simulink model "BD_PAR_AUTO_base_model"  (Simulink 10.3)
settings: Solver=ode1  StartTime=0.0  StopTime=max(cyc_mph(:,1))  FixedStep=1  MaxStep=1  RelTol=1e-3  AbsTol=1e-3
undefined symbols (not defined in the file): acc_dcdc_eff, acc_elec_eff, acc_elec_pwr, acc_mech_eff, acc_mech_pwr, acc_mech_trq, air_cp, amb_tmp, cs_charge_deplete_bool, cs_charge_trq, cs_electric_decel_spd, cs_electric_launch_spd_hi, cs_electric_launch_spd_lo, cs_hi_soc, cs_lo_soc, cs_min_trq_frac, cs_off_trq_frac, cyc_avg_time, cyc_cargo_mass, cyc_elevation_init, cyc_filter_bool, cyc_grade, cyc_mph, enable_sim_stop_distance, enable_sim_stop_max_spd, enable_sim_stop_speed, enable_sim_stop_time, enable_stop, enable_stop_fc, ess_cap_scale, ess_coulombic_eff, ess_init_soc, ess_max_ah_cap, ess_max_volts, ess_min_volts, ess_mod_airflow, ess_mod_cp, ess_mod_init_tmp, ess_module_mass, ess_module_num, ess_on, ess_r_chg, ess_r_dis, ess_res_scale_coef, ess_res_scale_fun, ess_set_tmp, ess_soc, ess_th_calc, ess_th_res_off, ess_th_res_on, ess_tmp, ess_voc, ex_calc, ex_cat_co_frac, ex_cat_ext_cp, ex_cat_ext_emisv, ex_cat_ext_init_tmp, ex_cat_ext_mass, ex_cat_ext_sarea, ex_cat_hc_frac ... (+168)
(part 5 of 15)

== system BD_PAR_AUTO_base_model/<vc> par auto/gearbox control for use w/ AT/est. engine trq and spd ==
  prev gear number : Inport
  " prev eta_gb" : Inport  Port=2
  gb_trq_out_r : Inport  Port=3
  gb_spd_out_r : Inport  Port=4
  Block NOTES : Subsystem
      mask Display: disp('Block\nNOTES')
  Constant2 : Constant  Value=[1 1]
  Constant5 : Constant  Value=0
  Demux : Demux  Outputs=2
      settings: DisplayOption=none
  K_adv : Subsystem
  Logical Operator : Logic
  Logical Operator1 : Logic  Operator=NOT  Inputs=1
  Memory : Memory
  Mux1 : Mux  Inputs=2
  Mux2 : Mux  Inputs=2
  Relational Operator1 : RelationalOperator  Operator=>  RndMeth=Nearest  InputSameDT=on
  SR Look-Up Table SR=wout/win : Lookup  InputValues=htc_k_adv  Table=htc_sr
  Saturation1 : Saturate  UpperLimit=1  LowerLimit=0.7
  Saturation2 : Saturate  UpperLimit=inf  LowerLimit=0
  Switch : Switch  Threshold=eps
  TR Look-Up Table TR=Tout/Tin : Lookup  InputValues=htc_k_adv  Table=htc_tr
  TR,SR : Mux  Inputs=2
  gear ratio1 : Lookup  InputValues=[1:length(gb_ratio)]  Table=gb_ratio
  ~eng trq and spd : Product  Inputs=*/  InputSameDT=on  RndMeth=Zero  SaturateOnIntegerOverflow=on  OutDataTypeStr=Inherit: Same as first input
  ~gb_spd_in_r : Product  InputSameDT=on  RndMeth=Zero  SaturateOnIntegerOverflow=on  OutDataTypeStr=Inherit: Same as first input
  ~gb_trq_in_r : Product  Inputs=//*  InputSameDT=on  RndMeth=Zero  SaturateOnIntegerOverflow=on  OutDataTypeStr=Inherit: Same as first input
  est eng trq (Nm) : Outport
  est eng spd (rad/s) : Outport  Port=2
  gb_spd_in_est (rad/s)1 : Outport  Port=3
  wires:
  gb_trq_out_r/1 -> ~gb_trq_in_r/3
  gb_spd_out_r/1 -> ~gb_spd_in_r/2
  gear ratio1/1 -> ~gb_trq_in_r/1, ~gb_spd_in_r/1
  TR,SR/1 -> Switch/1
  Constant2/1 -> Switch/3
  Switch/1 -> ~eng trq and spd/2
  " prev eta_gb"/1 -> Saturation1/1
  Saturation1/1 -> ~gb_trq_in_r/2
  Demux/2 -> Saturation2/1
  Saturation2/1 -> est eng spd (rad/s)/1
  Constant5/1 -> Relational Operator1/2
  Relational Operator1/1 -> Logical Operator/1
  prev gear number/1 -> gear ratio1/1
  Demux/1 -> est eng trq (Nm)/1
  Memory/1 -> Logical Operator1/1
  Logical Operator1/1 -> Logical Operator/2
  Logical Operator/1 -> Switch/2
  [locked_up] -> Memory/1
  Mux1/1 -> ~eng trq and spd/1
  ~eng trq and spd/1 -> Demux/1
  Mux2/1 -> K_adv/1("Req'd output trq and spd (Nm), (rad/s)")
  K_adv/1(K_adv) -> TR Look-Up Table TR=Tout/Tin/1, SR Look-Up Table SR=wout/win/1
  TR Look-Up Table TR=Tout/Tin/1 -> TR,SR/1
  SR Look-Up Table SR=wout/win/1 -> TR,SR/2
  ~gb_trq_in_r/1 -> Mux2/1, Mux1/1, Relational Operator1/1
  ~gb_spd_in_r/1 -> Mux1/2, gb_spd_in_est (rad/s)1/1, Mux2/2

== system BD_PAR_AUTO_base_model/<vc> par auto/gearbox control for use w/ AT/est. engine trq and spd assuming lockup ==
  new gear number : Inport
  " prev eta_gb" : Inport  Port=2
  gb_trq_out_r : Inport  Port=3
  gb_spd_in_est : Inport  Port=4
  Block NOTES : Subsystem
      mask Display: disp('Block\nNOTES')
  Memory : Memory  InitialCondition=gb_ratio(1)
  Saturation1 : Saturate  UpperLimit=1  LowerLimit=0.7
  Saturation2 : Saturate  UpperLimit=inf  LowerLimit=0
  gear ratio1 : Lookup  InputValues=[1:length(gb_ratio)]  Table=gb_ratio
  ~gb_spd_in_r : Product  Inputs=*/*  InputSameDT=on  RndMeth=Zero  SaturateOnIntegerOverflow=on  OutDataTypeStr=Inherit: Same as first input
  ~gb_trq_in_r : Product  Inputs=//*  InputSameDT=on  RndMeth=Zero  SaturateOnIntegerOverflow=on  OutDataTypeStr=Inherit: Same as first input
  est eng trq (Nm) : Outport
  est eng spd (rad/s) : Outport  Port=2
  wires:
  Saturation1/1 -> ~gb_trq_in_r/2
  " prev eta_gb"/1 -> Saturation1/1
  gear ratio1/1 -> ~gb_trq_in_r/1, ~gb_spd_in_r/1, Memory/1
  gb_trq_out_r/1 -> ~gb_trq_in_r/3
  new gear number/1 -> gear ratio1/1
  Saturation2/1 -> est eng spd (rad/s)/1
  Memory/1 -> ~gb_spd_in_r/2
  gb_spd_in_est/1 -> ~gb_spd_in_r/3
  ~gb_trq_in_r/1 -> est eng trq (Nm)/1
  ~gb_spd_in_r/1 -> Saturation2/1

== system BD_PAR_AUTO_base_model/<vc> par auto/gearbox control for use w/ AT/shifting1 ==
  gear number : Inport
  Constant : Constant  Value=gb_shift_delay-1e-6
  Relational Operator : RelationalOperator  Operator=<  RndMeth=Nearest  InputSameDT=on
  time since last shift : Subsystem
      mask Display: disp('time since\nlast shift')
  out_1 : Outport  InitialOutput=0
  wires:
  time since last shift/1(out_1) -> Relational Operator/1
  Constant/1 -> Relational Operator/2
  gear number/1 -> time since last shift/1(in_1)
  Relational Operator/1 -> out_1/1

== system BD_PAR_AUTO_base_model/<vc> par auto/gearbox control for use w/ AT/upshift  command ==
  prev gear number : Inport
  engine load : Inport  Port=2
  engine speed : Inport  Port=3
  Mux : Mux  Inputs=2
  Relational Operator : RelationalOperator  Operator=<  RndMeth=Nearest  InputSameDT=on
  load fraction : Subsystem  mask(Gear Selector){spd=gb_upshift_spd, load=gb_upshift_load}
      mask prompts: spd "Speeds:"; load "Load Fractions:"
      mask help:
      | This block will perform a linear interplation (extrapolation outside of bounds) to determine the shift point load fraction associated with the current gear number and speed.
      |
      | The Speeds parameter should be defined as an array of vectors containing speeds for each gear number.  The Load Fractions parameter should be defined as a array of vectors containing load fractions indexed by the speeds in the Speeds parameter for each gear number.
      mask Help:
      | Reference the base workspace variables - gb_**shift_spd and gb_**shift_load  where ** is either up for upshift conditions or dn for downshift conditions.
      | 
      | Or define the arrays as follows:
      | 
      | {[spd1 spd2 spd3 spd4]; [spd1 spd2 spd3 spd4]; ...}
      | 
      | {[load1 load2 load3 load4]; [load1 load2 load3 load4]; ...}
      | 
      | where each array contains one row for each gear in the gearbox.  Speeds should be defined in rad/s and loads as a decimal fraction.
  command : Outport  InitialOutput=0
  wires:
  load fraction/1(Out1) -> Relational Operator/2
  engine load/1 -> Relational Operator/1
  prev gear number/1 -> Mux/1
  Mux/1 -> load fraction/1(In1)
  engine speed/1 -> Mux/2
  Relational Operator/1 -> command/1

== system BD_PAR_AUTO_base_model/<vc> par auto/motor controller logic/Block NOTES ==
  note: This block models a motor/controller's logic, modulating the power input requirement as follows:
      | - enforcing the maximum current limit of the motor/controller
      | - shutting the motor off if the average speed over the time step ==0
      | - shutting the motor off if the transmission is shifting.

== system BD_PAR_AUTO_base_model/<vc> par auto/motor controller logic/Sign ==
  in_1 : Inport
  Constant : Constant  Value=0
  Relational Operator : RelationalOperator  Operator=>  RndMeth=Nearest  InputSameDT=on
  Relational Operator1 : RelationalOperator  Operator=<  RndMeth=Nearest  InputSameDT=on
  Sum : Sum  Inputs=+-  InputSameDT=on  SaturateOnIntegerOverflow=on  OutDataTypeStr=Inherit: Same as first input
  out_1 : Outport  InitialOutput=0
  wires:
  Sum/1 -> out_1/1
  Relational Operator/1 -> Sum/1
  Relational Operator1/1 -> Sum/2
  Constant/1 -> Relational Operator/2, Relational Operator1/2
  in_1/1 -> Relational Operator1/1, Relational Operator/1

== system BD_PAR_AUTO_base_model/<vc> par auto/parallel clutch control/Block NOTES ==
  note: This clutch control block determines the clutch state given the req'd clutch output torque
      | and speed (labelled as gearbox input torque and speed), and the gear number history.
      |                           conditions                                                                       clutch state
      | gear is being shifted OR (trq <~ 0 AND (engine is                                     1 == disengaged
      | clutched to avoid compression braking OR spd < idle))
      |
      | (trq >~ 0) AND (spd < launch speed) AND clutch                                       2 == slipping
      | was not engaged during previous time step
      |
      | neither of above sets of conditions are met                                          3 == engaged
      |
      | But the clutch is always disengaged when the engine is off or was off within the past 0.5 s.

== system BD_PAR_AUTO_base_model/<vc> par auto/parallel clutch control/gearbox speed estimator ==
  gb_spd_in_r if no gear change : Inport
  Block NOTES : Subsystem
      mask Display: disp('Block\nNOTES')
  Constant : Constant  Value=eps
  Constant1 : Constant  Value=0
  Constant2 : Constant
  Constant3 : Constant  Value=0.11
  Gain : Gain  Gain=0.447  SaturateOnIntegerOverflow=on  OutDataTypeStr=Inherit: Same as input  ParamDataTypeStr=Inherit: Same as input
  Logical : Logic
  Memory : Memory  InitialCondition=cyc_mph(1,2)*0.447/wh_radius*fd_ratio*gb_ratio(gb_num_init)
  Memory1 : Memory  InitialCondition=1
  Product : Product  Inputs=**/  InputSameDT=on  RndMeth=Zero  SaturateOnIntegerOverflow=on  OutDataTypeStr=Inherit: Same as first input
  Relational : RelationalOperator  Operator=>  RndMeth=Nearest  InputSameDT=on
  Relational1 : RelationalOperator  Operator=<=  RndMeth=Nearest  InputSameDT=on
  Sum : Sum  InputSameDT=on  SaturateOnIntegerOverflow=on  OutDataTypeStr=Inherit: Same as first input
  Sum1 : Sum  Inputs=-+  InputSameDT=on  SaturateOnIntegerOverflow=on  OutDataTypeStr=Inherit: Same as first input
  Switch : Switch  Threshold=eps
  Switch1 : Switch  Threshold=eps
  dt : Subsystem
  Out1 : Outport
  wires:
  Product/1 -> Switch/1
  Sum/1 -> Product/3
  Gain/1 -> Product/2
  [veh_spd_a_rec] -> Sum/1, Switch/2
  Constant1/1 -> Switch/3
  Memory/1 -> Switch1/1
  Constant/1 -> Sum/2
  [cyc_mph_r] -> Sum1/2
  [mpha] -> Gain/1, Sum1/1
  Constant2/1 -> Relational/2
  Sum1/1 -> Relational/1
  Relational/1 -> Memory1/1
  Switch/1 -> Memory/1
  Switch1/1 -> Out1/1
  gb_spd_in_r if no gear change/1 -> Switch1/3
  [gb_spd_in_a] -> Product/1
  Constant3/1 -> Relational1/2
  Relational1/1 -> Logical/2
  Memory1/1 -> Logical/1
  Logical/1 -> Switch1/2
  dt/1(Out1) -> Relational1/1

== system BD_PAR_AUTO_base_model/<vc> par auto/sim stop subsystem/Block NOTES ==
  note: This block controls the simulation stop time.  The simulation maybe
      | stop based on the achievement of a specified speed, a max speed, a time, a distance, or an engine condition.

== system BD_PAR_AUTO_base_model/<vc> par auto/sim stop subsystem/stop sim distance ==
  distance : Inport
  Enable : EnablePort
  Const : Constant  Value=sim_stop_distance
  Relational Operator2 : RelationalOperator  Operator=>  RndMeth=Nearest  InputSameDT=on
  Out1 : Outport  InitialOutput=0
  wires:
  Relational Operator2/1 -> Out1/1
  Const/1 -> Relational Operator2/2
  distance/1 -> Relational Operator2/1

== system BD_PAR_AUTO_base_model/<vc> par auto/sim stop subsystem/stop sim fc ==
  engine on? : Inport
  Enable : EnablePort
  Clock : Clock
  Const : Constant  Value=j17_endtimes
  Logical Operator : Logic
  Logical Operator1 : Logic  Operator=OR
  Logical Operator2 : Logic  Operator=OR  Inputs=1
  Manual Switch : ManualSwitch  CurrentSetting=0
  Memory : Memory
  Relational Operator : RelationalOperator  Operator===  RndMeth=Nearest  InputSameDT=on
  Relational Operator1 : RelationalOperator  RndMeth=Nearest  InputSameDT=on
  Out1 : Outport  InitialOutput=0
  wires:
  Logical Operator/1 -> Out1/1
  Logical Operator2/1 -> Logical Operator/2
  Logical Operator1/1 -> Logical Operator/1, Memory/1
  Memory/1 -> Logical Operator1/2
  engine on?/1 -> Logical Operator1/1
  Const/1 -> Relational Operator/2, Relational Operator1/2
  Clock/1 -> Relational Operator/1, Relational Operator1/1
  Relational Operator/1 -> Manual Switch/1
  Relational Operator1/1 -> Manual Switch/2
  Manual Switch/1 -> Logical Operator2/1

== system BD_PAR_AUTO_base_model/<vc> par auto/sim stop subsystem/stop sim max spd ==
  speed : Inport
  Enable : EnablePort
  Block NOTES : Subsystem
      mask Display: disp('Block\nNOTES')
  Const : Constant  Value=eps
  Logical Operator : Logic
  Relational Operator2 : RelationalOperator  Operator=>  RndMeth=Nearest  InputSameDT=on
  Relational Operator3 : RelationalOperator  Operator=<=  RndMeth=Nearest  InputSameDT=on
  Transport Delay : TransportDelay  DelayTime=(gb_shift_delay*5)+1
  Out1 : Outport  InitialOutput=0
  wires:
  Relational Operator3/1 -> Logical Operator/1
  Transport Delay/1 -> Relational Operator3/2
  speed/1 -> Transport Delay/1, Relational Operator2/1, Relational Operator3/1
  Logical Operator/1 -> Out1/1
  Relational Operator2/1 -> Logical Operator/2
  Const/1 -> Relational Operator2/2

== system BD_PAR_AUTO_base_model/<vc> par auto/sim stop subsystem/stop sim speed ==
  speed : Inport
  Enable : EnablePort
  Const : Constant  Value=sim_stop_speed
  Relational Operator2 : RelationalOperator  Operator=>  RndMeth=Nearest  InputSameDT=on
  Out1 : Outport  InitialOutput=0
  wires:
  speed/1 -> Relational Operator2/1
  Const/1 -> Relational Operator2/2
  Relational Operator2/1 -> Out1/1

== system BD_PAR_AUTO_base_model/<vc> par auto/sim stop subsystem/stop sim time ==
  time : Inport
  Enable : EnablePort
  Const : Constant  Value=sim_stop_time
  Relational Operator2 : RelationalOperator  Operator=>  RndMeth=Nearest  InputSameDT=on
  Out1 : Outport  InitialOutput=0
  wires:
  Relational Operator2/1 -> Out1/1
  Const/1 -> Relational Operator2/2
  time/1 -> Relational Operator2/1

== system BD_PAR_AUTO_base_model/drive cycle <cyc>/distance travelled (m)/Block NOTES ==
  note: This block calculates the distance travelled by the
      |  vehicle based on the achieved speed.

== system BD_PAR_AUTO_base_model/drive cycle <cyc>/super-smooth, no-lag trace/Subsystem ==
  in_1 : Inport
  Constant1 : Constant  Value=n
  Integrator : Integrator
  Product : Product  Inputs=*/  InputSameDT=on  RndMeth=Zero  SaturateOnIntegerOverflow=on  OutDataTypeStr=Inherit: Same as first input
  Sum : Sum  Inputs=+-  InputSameDT=on  SaturateOnIntegerOverflow=on  OutDataTypeStr=Inherit: Same as first input
  Transport Delay : TransportDelay  DelayTime=n
  out_1 : Outport  InitialOutput=0
  wires:
  Integrator/1 -> Sum/1, Transport Delay/1
  Transport Delay/1 -> Sum/2
  Sum/1 -> Product/1
  in_1/1 -> Integrator/1
  Product/1 -> out_1/1
  Constant1/1 -> Product/2

== system BD_PAR_AUTO_base_model/drive cycle <cyc>/super-smooth, no-lag trace/repeated cycle ==
  Clock : Clock
  Fcn1 : Fcn  Expr=rem(u+avgtime*0.75,period)
  Look-Up Table : Lookup  InputValues=t  Table=y
  out_1 : Outport  InitialOutput=0
  wires:
  Fcn1/1 -> Look-Up Table/1
  Clock/1 -> Fcn1/1
  Look-Up Table/1 -> out_1/1

== system BD_PAR_AUTO_base_model/electric acc loads <acc>/Electrical Accessory Loads v2 <acc>/Accessory SDO ==
  data bus : Inport
  Demux : Demux  Outputs=3
      settings: DisplayOption=none
  To Workspace : ToWorkspace  VariableName=acc_elec_pwr_r  SampleTime=-1
  To Workspace3 : ToWorkspace  VariableName=acc_elec_pwr_a  SampleTime=-1
  To Workspace4 : ToWorkspace  VariableName=acc_elec_pwr_est  SampleTime=-1
  electrical power logging : Subsystem  mask{eff=acc_mech_eff}
      mask prompts: eff "efficiency of accessory systems (decimal)"
  wires:
  Demux/3 -> To Workspace4/1
  Demux/2 -> electrical power logging/1(In1), To Workspace3/1
  Demux/1 -> To Workspace/1
  data bus/1 -> Demux/1

== system BD_PAR_AUTO_base_model/electric acc loads <acc>/Electrical Accessory Loads v2 <acc>/Block NOTES ==
  note: This is the electrical auxiliary loads model.
  note: In terms of an interface, the model assumes electrical power generated from
      | a powersource (or powersources)
      |
      | This model takes in requested driveline electrical power output requests and
      | augments power to account for electrically driven accessories.
      |
      | The power passed along down to the driveline is only power to move the
      | vehicle.

== system BD_PAR_AUTO_base_model/electric acc loads <acc>/Electrical Accessory Loads v2 <acc>/backward model ==
  note: Power Electrical
      | Accessory
      | (W)
  note: P, W, for driveline
  note: Pwr, W, powersource out
  pwr_in : Inport
  on/off : Inport  Port=2
  Constant : Constant  Value=load_on
  Product : Product  Inputs=***  InputSameDT=on  RndMeth=Zero  SaturateOnIntegerOverflow=on  OutDataTypeStr=Inherit: Same as first input
  Sum : Sum  Inputs=|++  InputSameDT=on  SaturateOnIntegerOverflow=on  OutDataTypeStr=Inherit: Same as first input
  electrical accessories (W) : Subsystem  BlockChoice=Electrical Accessories: Time Variable
      settings: AttributesFormatString=%<BlockChoice>  TemplateBlock=lib_accessory/electrical accessories (W)  MemberBlocks=Electrical Accessories: Constant,Electrical Accessories: Time Variable
      mask Display: image(imread('bdi_acc_elec_cs.bmp'))
  elec_out : Outport
  elec_acc_out : Outport  Port=2
  wires:
  Product/1 -> Sum/2, elec_acc_out/1
  Constant/1 -> Product/3
  on/off/1 -> Product/2
  electrical accessories (W)/1(P_elec_acc) -> Product/1
  pwr_in/1 -> Sum/1
  Sum/1 -> elec_out/1

== system BD_PAR_AUTO_base_model/electric acc loads <acc>/Electrical Accessory Loads v2 <acc>/forward model ==
  note: ASSUMPTIONS
  note: This calculation assumes that the power provider is never so power limited as to
      | not be able to provide at least the value of acc_pwr_in.
  note: electric
      | accessory
      | power (W)
  note: Power Available
  note: Power to driveline
  pwr_in : Inport
  acc_pwr_in : Inport  Port=2
  Sum : Sum  Inputs=|+-  InputSameDT=on  SaturateOnIntegerOverflow=on  OutDataTypeStr=Inherit: Same as first input
  pwr_out : Outport
  acc_pwr_out : Outport  Port=2
  wires:
  acc_pwr_in/1 -> acc_pwr_out/1, Sum/2
  pwr_in/1 -> Sum/1
  Sum/1 -> pwr_out/1

== system BD_PAR_AUTO_base_model/energy storage <ess>/ess config/energy storage <ess> ==
  power req'd into bus (W) : Inport
  Block NOTES : Subsystem
      mask Display: disp('Block\nNOTES')
  Const : Constant  Value=enable_stop
  Fcn : Fcn  Expr=u[1]*u[1]*u[2]*(u[1]>=0)+u[1]*u[1]*u[2]*u(4)*u(4)*(u[1]<0)-u[1]*u[3]*(1-u(4))*(u[1]<0)
  Memory : Memory  InitialCondition=ess_mod_init_tmp
  Mux : Mux
  Product : Product  InputSameDT=on  RndMeth=Zero  SaturateOnIntegerOverflow=on  OutDataTypeStr=Inherit: Same as first input
  SOC algorithm : Subsystem
  To WS1 : ToWorkspace  VariableName=ess_pwr_loss_a
  To WS2 : ToWorkspace  VariableName=ess_mod_tmp
  To WS3 : ToWorkspace  VariableName=ess_air_tmp
  To WS4 : ToWorkspace  VariableName=ess_air_th_pwr
  To Workspace8 : ToWorkspace  VariableName=ess_pwr_out_r  SampleTime=-1
  To Workspace9 : ToWorkspace  VariableName=ess_pwr_out_a  SampleTime=-1
  compute current : Subsystem
  coul eff : Lookup  InputValues=ess_tmp  Table=ess_coulombic_eff
  do ex calcs? : Constant  Value=ess_th_calc
  documentation9 : Subsystem
      settings: OpenFcn=web(['file:\\\' which('energy_storage.htm')]);
      mask Display: image(imread('doc_man.jpg'))
  ess tmp : Subsystem  TreatAsAtomicUnit=on
  limit power : Subsystem
  max pack pwr (W)1 : Subsystem
  "pack Voc, Rint" : Subsystem
  stop sim : Subsystem  TreatAsAtomicUnit=on
  power available to bus (W) : Outport  InitialOutput=0
  tag scope: SOC=global, bus_voltage=global, ess_max_chg_pwr=global, ess_max_pwr=global, ess_pwr_out_a=global, ess_tmp=global
  wires:
  max pack pwr (W)1/2(max ess charge pwr) -> [ess_max_chg_pwr]
  Memory/1 -> [ess_tmp], max pack pwr (W)1/2(ess_mod_tmp), "pack Voc, Rint"/3(mod tmp   (C)), coul eff/1, SOC algorithm/2(tmp (C)), To WS2/1
  max pack pwr (W)1/1(max ess discharge pwr) -> [ess_max_pwr]
  coul eff/1 -> Mux/4
  ess tmp/1(Tess) -> Memory/1
  ess tmp/3(Qair) -> To WS4/1
  ess tmp/2(Tair) -> To WS3/1
  limit power/1("Pbty, limited") -> compute current/3(limited output power (W))
  "pack Voc, Rint"/1(pack open- circuit voltage) -> limit power/3(Voc), compute current/1(Voc)
  "pack Voc, Rint"/2(pack resistance) -> Mux/2, limit power/4(Rint), compute current/2(Rint)
  Const/1 -> stop sim/Enable
  SOC algorithm/1(SOC1) -> max pack pwr (W)1/1(SOC), limit power/1(SOC), "pack Voc, Rint"/1(SOC (prev)), [SOC], stop sim/1(SOC)
  do ex calcs?/1 -> ess tmp/Enable
  Fcn/1 -> ess tmp/1(Qess_gen), To WS1/1
  Product/1 -> [ess_pwr_out_a], To Workspace9/1, power available to bus (W)/1
  compute current/1(I_) -> Mux/1, Product/1, SOC algorithm/1((A))
  power req'd into bus (W)/1 -> "pack Voc, Rint"/2(req'd battery power (W)), limit power/2(Pbty), To Workspace8/1
  Mux/1 -> Fcn/1
  compute current/2(V_) -> [bus_voltage], Mux/3, Product/2

== system BD_PAR_AUTO_base_model/exhaust sys <ex>/ex gas heat flow/Block NOTES ==
  note: EXHAUST GAS HEAT TRANSFER
      | This block models the heat loss from the exhaust gas as it flows from the engine through the manifold,
      | downpipe, and catalytic converter.  Also included is the increase in gas temperature within the converter
      | due to the catalysis of HC, CO, and NOx. The block is conditionally executed only if engine_on=1.

== system BD_PAR_AUTO_base_model/exhaust sys <ex>/ex gas heat flow/converter ==
  h,exg : Inport
  Cexg : Inport  Port=2
  Texgi : Inport  Port=3
  Tex : Inport  Port=4
  " Q/C" : Product  Inputs=/*  SaturateOnIntegerOverflow=on
  1/A : Gain  Gain=1/(ex_cat_moni_sarea+ex_cat_int_sarea-ex_cat_mon_sarea)  SaturateOnIntegerOverflow=on
  Demux3 : Demux  Outputs=2
  MinMax : MinMax  Inputs=2
  Mux16 : Mux
  Qci2g_ : Fcn  Expr=u(1)*(ex_cat_int_sarea - ex_cat_mon_sarea)*(u(3)-u(4))
  Qcm2g_ : Fcn  Expr=u(1)*ex_cat_moni_sarea*(u(2)-u(4))
  Selector3 : Selector  InputPortWidth=5  IndexOptions=Index vector (dialog)  Indices=[ 1 2 ]  OutputSizes=1
  T : Sum  SaturateOnIntegerOverflow=on
  T1 : Sum  SaturateOnIntegerOverflow=on
  Texgo : Outport  OutputWhenDisabled=reset  InitialOutput=amb_tmp
  Qcm2g : Outport  Port=2  OutputWhenDisabled=reset  InitialOutput=0
  Qci2g : Outport  Port=3  OutputWhenDisabled=reset  InitialOutput=0
  wires:
  Cexg/1 -> " Q/C"/1, 1/A/1
  h,exg/1 -> MinMax/2
  1/A/1 -> MinMax/1
  MinMax/1 -> Mux16/1
  Tex/1 -> Selector3/1
  Selector3/1 -> Demux3/1
  Demux3/1 -> Mux16/2
  Demux3/2 -> Mux16/3
  Texgi/1 -> T/2, Mux16/4
  Mux16/1 -> Qcm2g_/1, Qci2g_/1
  Qci2g_/1 -> T1/2, Qci2g/1
  Qcm2g_/1 -> T1/1, Qcm2g/1
  " Q/C"/1 -> T/1
  T1/1 -> " Q/C"/2
  T/1 -> Texgo/1

== system BD_PAR_AUTO_base_model/exhaust sys <ex>/ex gas heat flow/inlet pipe ==
  h,exg : Inport
  Cexg : Inport  Port=2
  Texgi : Inport  Port=3
  Tex : Inport  Port=4
  " Q/C" : Product  Inputs=/*  SaturateOnIntegerOverflow=on
  A : Gain  Gain=ex_cat_pipe_sarea  SaturateOnIntegerOverflow=on
  Memory : Memory  InitialCondition=cyc_mph(1,2)*.447
  MinMax : MinMax  Inputs=2
  Mux19 : Mux  Inputs=3
  Selector2 : Selector  InputPortWidth=5  IndexOptions=Index vector (dialog)  Indices=3  OutputSizes=1
  T : Sum  SaturateOnIntegerOverflow=on
  Ts-Tex,ave : Fcn  Expr=u(2) - (u(3)+u(1))/2
  tailpipe  emis : Product  SaturateOnIntegerOverflow=on
  Texgo : Outport  OutputWhenDisabled=reset  InitialOutput=amb_tmp
  tag scope: Qp2g=global, Tgpo=global
  wires:
  h,exg/1 -> A/1
  MinMax/1 -> tailpipe  emis/1
  A/1 -> MinMax/2
  Cexg/1 -> MinMax/1, " Q/C"/1
  tailpipe  emis/1 -> " Q/C"/2, [Qp2g]
  " Q/C"/1 -> T/1
  Texgi/1 -> T/2, Mux19/1
  T/1 -> Texgo/1, [Tgpo], Memory/1
  Tex/1 -> Selector2/1
  Mux19/1 -> Ts-Tex,ave/1
  Ts-Tex,ave/1 -> tailpipe  emis/2
  Selector2/1 -> Mux19/2
  Memory/1 -> Mux19/3

== system BD_PAR_AUTO_base_model/exhaust sys <ex>/ex gas heat flow/manifold  ==
  h,exg : Inport
  Cexg : Inport  Port=2
  Texgi : Inport  Port=3
  Tex : Inport  Port=4
  " Q/C" : Product  Inputs=/*  SaturateOnIntegerOverflow=on
  A : Gain  Gain=ex_manif_sarea  SaturateOnIntegerOverflow=on
  Memory : Memory  InitialCondition=cyc_mph(1,2)*.447
  MinMax : MinMax  Inputs=2
  Mux19 : Mux  Inputs=3
  Selector1 : Selector  InputPortWidth=5  IndexOptions=Index vector (dialog)  Indices=5  OutputSizes=1
  T : Sum  SaturateOnIntegerOverflow=on
  Ts-Tex,ave : Fcn  Expr=u(2) - (u(3)+u(1))/2
  tailpipe  emis : Product  SaturateOnIntegerOverflow=on
  Texgo : Outport  OutputWhenDisabled=reset  InitialOutput=amb_tmp
  tag scope: Qma2g=global, Tgmo=global
  wires:
  h,exg/1 -> A/1
  MinMax/1 -> tailpipe  emis/1
  A/1 -> MinMax/2
  Cexg/1 -> MinMax/1, " Q/C"/1
  " Q/C"/1 -> T/1
  T/1 -> [Tgmo], Texgo/1, Memory/1
  tailpipe  emis/1 -> " Q/C"/2, [Qma2g]
  Tex/1 -> Selector1/1
  Selector1/1 -> Mux19/2
  Mux19/1 -> Ts-Tex,ave/1
  Memory/1 -> Mux19/3
  Ts-Tex,ave/1 -> tailpipe  emis/2
  Texgi/1 -> Mux19/1, T/2

== system BD_PAR_AUTO_base_model/exhaust sys <ex>/ex sys heat flow/Block NOTES ==
  note: CATALYTIC CONVERTER HEAT LOSS
      | This block models the heat loss from a catalytic converter (conventional or vacuum-insulated).
      | Convection (as a function of vehicle speed), radiation, and conduction effects are included.
      | Converter monolith (m), interior (i), pipe (p), and exterior (x) and engine manifold
      | heat flows are estimated based on the temperatures from the previous iteration.

== system BD_PAR_AUTO_base_model/exhaust sys <ex>/removal efficiencies/removal efficiencies (base ADVISOR) ==
  Ex Cat T (C) : Inport
  Enable : EnablePort  StatesWhenEnabling=reset
  CO temp eff : Lookup  InputValues=ex_cat_tmp_range  Table=ex_cat_co_frac
  HC temp eff : Lookup  InputValues=ex_cat_tmp_range  Table=ex_cat_hc_frac
  Mux : Mux
  NOx temp eff : Lookup  InputValues=ex_cat_tmp_range  Table=ex_cat_nox_frac
  PM temp eff : Lookup  InputValues=ex_cat_tmp_range  Table=ex_cat_pm_frac
  removal effs : Outport  OutputWhenDisabled=reset  InitialOutput=0
  wires:
  Ex Cat T (C)/1 -> PM temp eff/1, NOx temp eff/1, CO temp eff/1, HC temp eff/1
  Mux/1 -> removal effs/1
  PM temp eff/1 -> Mux/4
  NOx temp eff/1 -> Mux/3
  HC temp eff/1 -> Mux/1
  CO temp eff/1 -> Mux/2

== system BD_PAR_AUTO_base_model/exhaust sys <ex>/removal efficiencies/removal efficiencies ORNL ==
  gas_flow (g/s) : Inport
  Ex Gas T (C) : Inport  Port=2
  O2_exh (g/s) : Inport  Port=3
  emis Engine Out (g/s) : Inport  Port=4
  Ex Cat T (C) : Inport  Port=5
  Enable : EnablePort  StatesWhenEnabling=reset
  CO : Terminator
  CO-Conversion : Subsystem
  Constant : Constant  Value=1200
  Demux : Demux
  HC-Conversion : Subsystem
  Mux : Mux
  NOx_Eff : Subsystem
  PM : Terminator
  PM temp eff : Lookup  InputValues=ex_cat_tmp_range  Table=ex_cat_pm_frac
  Product : Product  Inputs=/*  SaturateOnIntegerOverflow=on
  Volume  Flow (m^3/sec) : Gain  Gain=2.96E6  SaturateOnIntegerOverflow=on
  removal effs : Outport  OutputWhenDisabled=reset  InitialOutput=0
  wires:
  Mux/1 -> removal effs/1
  gas_flow (g/s)/1 -> CO-Conversion/4(ex_gas_flow), HC-Conversion/4(ex_gas_flow), Product/2
  Ex Cat T (C)/1 -> PM temp eff/1
  O2_exh (g/s)/1 -> CO-Conversion/3(O2_exh), HC-Conversion/3(O2_exh)
  CO-Conversion/1(CO_eff) -> Mux/2
  HC-Conversion/1(HC_eff) -> Mux/1
  NOx_Eff/1(NOx_eff) -> Mux/3
  PM temp eff/1 -> Mux/4
  Ex Gas T (C)/1 -> NOx_Eff/2(Ex_temp), CO-Conversion/2(T_exh), HC-Conversion/2(T_exh)
  Volume  Flow (m^3/sec)/1 -> NOx_Eff/1(vol_flow), CO-Conversion/1(vol_flow), HC-Conversion/1(vol_flow)
  Demux/1 -> NOx_Eff/3(HC_Inlet)
  Demux/3 -> NOx_Eff/4(NOx_Inlet)
  Demux/2 -> CO/1
  Demux/4 -> PM/1
  emis Engine Out (g/s)/1 -> Demux/1
  Constant/1 -> Product/1
  Product/1 -> Volume  Flow (m^3/sec)/1

== system BD_PAR_AUTO_base_model/fuel converter  <fc>/engine speed estimator/Block NOTES ==
  note: If the clutch is engaged and the trace was missed in the previous time step:
      | The estimated engine speed for the current time step is the actual engine
      | speed from the previous time step.
      |
      | If the clutch is disengaged and the speed is commanded to increase (spin up):
      | The engine speed is the lesser of the commanded speed and the maximum
      | speed attainable given the engine capability.
      |
      | If the clutch is disengaged at the speed is commanded to decrease (spin down):
      | The engine speed is computed by integrating with respect to time the ratio of
      |  closed-throttle torque to engine inertia.
      |
      | Otherwise:
      | The engine speed is equal to the speed command, but no greater than the
      | engine's maximum speed nor less than the engine's idle speed (if the engine is on.)

== system BD_PAR_AUTO_base_model/fuel converter  <fc>/engine speed estimator/dt ==
  Clock : Clock
  Memory1 : Memory  InitialCondition=-0.1
  Sum1 : Sum  Inputs=+-  InputSameDT=on  SaturateOnIntegerOverflow=on  OutDataTypeStr=Inherit: Same as first input
  out_1 : Outport  InitialOutput=0
  wires:
  Sum1/1 -> out_1/1
  Memory1/1 -> Sum1/2
  Clock/1 -> Memory1/1, Sum1/1

== system BD_PAR_AUTO_base_model/fuel converter  <fc>/engine speed estimator/effect of inertia (Nm) ==
  req'd spd (rad/s) : Inport
  prev spd : Inport  Port=2
  Clock : Clock
  Constant : Constant  Value=fc_inertia
  Memory : Memory  InitialCondition=-0.1
  Product1 : Product  Inputs=**/  InputSameDT=on  RndMeth=Zero  SaturateOnIntegerOverflow=on  OutDataTypeStr=Inherit: Same as first input
  Sum : Sum  Inputs=+-  InputSameDT=on  SaturateOnIntegerOverflow=on  OutDataTypeStr=Inherit: Same as first input
  Sum1 : Sum  Inputs=+-  InputSameDT=on  SaturateOnIntegerOverflow=on  OutDataTypeStr=Inherit: Same as first input
  (Nm) : Outport  InitialOutput=0
  wires:
  Constant/1 -> Product1/1
  Clock/1 -> Sum1/1, Memory/1
  Memory/1 -> Sum1/2
  Product1/1 -> (Nm)/1
  prev spd/1 -> Sum/2
  req'd spd (rad/s)/1 -> Sum/1
  Sum1/1 -> Product1/3
  Sum/1 -> Product1/2

== system BD_PAR_AUTO_base_model/fuel converter  <fc>/engine speed estimator/just started spin-down/spin-up ==
  state : Inport
  Logical Operator : Logic
  Logical Operator1 : Logic  Operator=NOT  Inputs=1
  Memory1 : Memory  InitialCondition=1
  trigger : Outport  InitialOutput=0
  wires:
  state/1 -> Memory1/1, Logical Operator/1
  Logical Operator/1 -> trigger/1
  Logical Operator1/1 -> Logical Operator/2
  Memory1/1 -> Logical Operator1/1

== system BD_PAR_AUTO_base_model/fuel converter  <fc>/engine speed estimator/no-lag Reset Integrator ==
  in_1 : Inport
  in_2 : Inport  Port=2
  in_3 : Inport  Port=3
  Constant : Constant  Value=0
  Memory : Memory  InitialCondition=initval
  Product : Product  InputSameDT=on  RndMeth=Zero  SaturateOnIntegerOverflow=on  OutDataTypeStr=Inherit: Same as first input
  Sum : Sum  InputSameDT=on  SaturateOnIntegerOverflow=on  OutDataTypeStr=Inherit: Same as first input
  Switch : Switch  Threshold=eps
  dt : Subsystem
  in_2==0 : RelationalOperator  Operator===  RndMeth=Nearest  InputSameDT=on
  out_1 : Outport  InitialOutput=0
  wires:
  Constant/1 -> in_2==0/2
  in_2==0/1 -> Switch/2
  Switch/1 -> Memory/1, out_1/1
  Sum/1 -> Switch/1
  Memory/1 -> Sum/1
  Product/1 -> Sum/2
  dt/1(out_1) -> Product/1
  in_1/1 -> Product/2
  in_2/1 -> in_2==0/1
  in_3/1 -> Switch/3

== system BD_PAR_AUTO_base_model/fuel converter  <fc>/engine torque/Block NOTES ==
  note: If the engine is not spinning down with the clutch disengaged:
      | 1.  Engine brake (aka map) torque is given by the required shaft
      | torque plus enough torque to accelerate the engine's rotating
      | parts as commanded and torque to power the accessories,
      | subject to the engine's torque limits at the current speed.
      | 2.  Shaft torque is engine brake torque less the effects of inertia
      | and accessories.
      |
      | If the engine is spinning down:
      | 1.  Engine brake/map torque is the closed-throttle torque.
      | 2.  Shaft torque is zero.

== system BD_PAR_AUTO_base_model/fuel converter  <fc>/engine torque/T_closed throttle ==
  w_APU : Inport
  Saturation : Saturate  UpperLimit=max(fc_map_spd)*fc_spd_scale  LowerLimit=min(fc_map_spd)*fc_spd_scale
  ctt lookup : Lookup  InputValues=fc_map_spd*fc_spd_scale  Table=fc_ct_trq*fc_trq_scale
  T_closed throttle : Outport  InitialOutput=0
  wires:
  w_APU/1 -> Saturation/1
  Saturation/1 -> ctt lookup/1
  ctt lookup/1 -> T_closed throttle/1

== system BD_PAR_AUTO_base_model/fuel converter  <fc>/engine torque/T_max ==
  w_APU : Inport
  Saturation1 : Saturate  UpperLimit=max(fc_map_spd)*fc_spd_scale  LowerLimit=min(fc_map_spd)*fc_spd_scale
  max_torque lookup : Lookup  InputValues=fc_map_spd*fc_spd_scale  Table=fc_max_trq*fc_trq_scale
  T_max : Outport  InitialOutput=0
  tag scope: engine_rpm=global
  wires:
  Saturation1/1 -> [engine_rpm], max_torque lookup/1
  max_torque lookup/1 -> T_max/1
  w_APU/1 -> Saturation1/1

== system BD_PAR_AUTO_base_model/fuel converter  <fc>/engine torque/effect of inertia (Nm) ==
  engine spd (rad/s) : Inport
  >=0 : Saturate  UpperLimit=inf  LowerLimit=0
  Block NOTES : Subsystem
      mask Display: disp('Block\nNOTES')
  Clock : Clock
  Constant : Constant  Value=fc_inertia
  Constant1 : Constant  Value=max(fc_max_trq)*fc_trq_scale
  Constant2 : Constant  Value=0.01
  Memory : Memory  InitialCondition=-0.1
  Memory1 : Memory  InitialCondition=vc_idle_spd*vc_key_on(1,2)
  Memory2 : Memory
  MinMax : MinMax  Inputs=2  InputSameDT=on  SaturateOnIntegerOverflow=on
  Product : Product  InputSameDT=on  RndMeth=Zero  SaturateOnIntegerOverflow=on  OutDataTypeStr=Inherit: Same as first input
  Product1 : Product  Inputs=*/*  InputSameDT=on  RndMeth=Zero  SaturateOnIntegerOverflow=on  OutDataTypeStr=Inherit: Same as first input
  Relational : RelationalOperator  Operator=>  RndMeth=Nearest  InputSameDT=on
  Sum : Sum  Inputs=+-  InputSameDT=on  SaturateOnIntegerOverflow=on  OutDataTypeStr=Inherit: Same as first input
  Sum1 : Sum  Inputs=+-  InputSameDT=on  SaturateOnIntegerOverflow=on  OutDataTypeStr=Inherit: Same as first input
  Sum2 : Sum  Inputs=-+  InputSameDT=on  SaturateOnIntegerOverflow=on  OutDataTypeStr=Inherit: Same as first input
  Switch : Switch  Threshold=eps
  engine inertia as a function of total vehicle inertia (generous approximation) : Subsystem
  (Nm) : Outport  InitialOutput=0
  wires:
  engine spd (rad/s)/1 -> Sum/1, Memory1/1
  Constant2/1 -> Relational/2
  Sum2/1 -> Relational/1
  >=0/1 -> Switch/1
  Relational/1 -> Memory2/1
  Memory2/1 -> Switch/2
  Clock/1 -> Sum1/1, Memory/1
  Memory/1 -> Sum1/2
  Constant/1 -> Product1/3
  Sum1/1 -> Product1/2
  Switch/1 -> Product1/1
  [mpha] -> Sum2/1
  [cyc_mph_r] -> Sum2/2
  MinMax/1 -> (Nm)/1
  Product1/1 -> MinMax/2
  engine inertia as a function of total vehicle inertia (generous approximation)/1(Out1) -> Product/1
  Constant1/1 -> Product/2
  Product/1 -> MinMax/1
  Memory1/1 -> Sum/2
  Sum/1 -> Switch/3, >=0/1

== system BD_PAR_AUTO_base_model/fuel converter  <fc>/fuel use and EO emis Configurable Subsystem/fuel use and EO emis ==
  T (Nm) : Inport
  w (rad/s) : Inport  Port=2
  (gal/s) : Gain  Gain=1/fc_fuel_den*61.02/231  SaturateOnIntegerOverflow=on  OutDataTypeStr=Inherit: Same as input  ParamDataTypeStr=Inherit: Same as input
  Block NOTES : Subsystem
      mask Display: disp('Block\nNOTES')
  Demux : Demux  Outputs=2
      settings: DisplayOption=none
  "HOT engine maps " : Subsystem  TreatAsAtomicUnit=on
  Integrator : Integrator
  Mux4 : Mux  Inputs=[1 4 1 1 1]
  Mux5 : Mux  Inputs=[1 4 ]
  Selector3 : Selector  InputPortWidth=4  IndexOptions=Index vector (dialog)  Indices=2  OutputSizes=1
  Terminator : Terminator
  To Workspace10 : ToWorkspace  VariableName=fc_ex_gas_flow  SampleTime=-1
  To Workspace11 : ToWorkspace  VariableName=fc_ex_gas_tmp  SampleTime=-1
  To Workspace12 : ToWorkspace  VariableName=fc_ex_th_pwr  SampleTime=-1
  To Workspace13 : ToWorkspace  VariableName=fc_r_th_pwr  SampleTime=-1
  To Workspace14 : ToWorkspace  VariableName=fc_tmp  SampleTime=-1
  To Workspace16 : ToWorkspace  VariableName=fc_th_pwr  SampleTime=-1
  To Workspace17 : ToWorkspace  VariableName=fc_h_th_pwr  SampleTime=-1
  To Workspace18 : ToWorkspace  VariableName=fc_o2_flow  SampleTime=-1
  To Workspace19 : ToWorkspace  VariableName=fc_fuel_rate  SampleTime=-1
  To Workspace8 : ToWorkspace  VariableName=fc_emis_eo  SampleTime=-1
  To Workspace9 : ToWorkspace  VariableName=fc_clt_tmp  SampleTime=-1
  fc temp : Subsystem
  fc temp correct : Subsystem  TreatAsAtomicUnit=on
  cumulative fuel  use (gal) : Outport  InitialOutput=0
  "FC ON?, EOem, MFex, Tex, O2ex" : Outport  Port=2  InitialOutput=0
  Vv,Tfc : Outport  Port=3  InitialOutput=0
  tag scope: fc_clt_tmp=global
  wires:
  fc temp correct/1(fuel use (g/s)) -> To Workspace19/1, (gal/s)/1
  "HOT engine maps "/6(O2 exhaust (g/s)) -> To Workspace18/1, Mux4/5
  T (Nm)/1 -> fc temp correct/4(T (Nm)), "HOT engine maps "/1(T (Nm))
  w (rad/s)/1 -> fc temp correct/5(w (rad/s)), "HOT engine maps "/2(w (rad/s))
  Mux4/1 -> "FC ON?, EOem, MFex, Tex, O2ex"/1
  Mux5/1 -> Vv,Tfc/1
  [v_prev] -> Mux5/1, fc temp/1(veh spd (m/s))
  "HOT engine maps "/4(Ex Gas Flow (g/s)) -> Mux4/3, To Workspace10/1
  "HOT engine maps "/5(Ex Gas Temp (C)) -> Mux4/4, To Workspace11/1
  Integrator/1 -> cumulative fuel  use (gal)/1
  (gal/s)/1 -> Integrator/1
  "HOT engine maps "/2(HOT fuel use (g/s)) -> fc temp correct/2(HOT fuel use (g/s))
  "HOT engine maps "/3(HOT emis (g/s)) -> fc temp correct/3(HOT emis (g/s))
  fc temp/3(Tfc  (C)) -> Selector3/1, To Workspace14/1, Mux5/2
  fc temp/1(Tfc_old  (C)) -> Terminator/1
  "HOT engine maps "/7(ex heat (W)) -> To Workspace12/1
  Selector3/1 -> [fc_clt_tmp], To Workspace9/1, fc temp correct/1(Coolant T (C))
  "HOT engine maps "/1(fc heat (W)) -> fc temp/4(Qfc (W)), To Workspace16/1
  fc temp/2(Qfc r,h) -> Demux/1
  Demux/1 -> To Workspace13/1
  Demux/2 -> To Workspace17/1
  fc temp correct/2(EO emis (g/s)) -> Mux4/2, To Workspace8/1
  [engine_on] -> Mux4/1, fc temp correct/Enable, fc temp/3(fc ON?), "HOT engine maps "/Enable
  [key_on] -> fc temp/2(key ON?)

== system BD_PAR_AUTO_base_model/gearbox <gb>/Pout/Pin, neglecting inertia/Pout/Pin (neglecting inertia) ==
  in_1 : Inport
  in_2 : Inport  Port=2
  Fcn : Fcn  Expr=1/u
  Product : Product  SaturateOnIntegerOverflow=on
  out_1 : Outport  InitialOutput=0
  wires:
  in_1/1 -> Product/1
  Fcn/1 -> Product/2
  Product/1 -> out_1/1
  in_2/1 -> Fcn/1

== system BD_PAR_AUTO_base_model/gearbox <gb>/Pout/Pin, neglecting inertia/make division bombproof ==
  note: only add eps if Tin-Tinertia is == 0 (this avoids problems when Tin-Tineratia == -eps
      | which happens from time to time
  Tin-Tinertia : Inport
  Block NOTES : Subsystem
      mask Display: disp('Block\nNOTES')
  Constant : Constant  Value=eps
  Constant1 : Constant  Value=0
  Product : Product  SaturateOnIntegerOverflow=on
  Relational Operator1 : RelationalOperator  Operator===  RndMeth=Nearest  InputSameDT=on
  make division bombproof : Sum  SaturateOnIntegerOverflow=on
  Out1 : Outport
  wires:
  Tin-Tinertia/1 -> make division bombproof/1, Relational Operator1/1
  Constant1/1 -> Relational Operator1/2
  Product/1 -> make division bombproof/2
  Relational Operator1/1 -> Product/1
  Constant/1 -> Product/2
  make division bombproof/1 -> Out1/1

== system BD_PAR_AUTO_base_model/gearbox <gb>/loss (Nm)/3D discrete lookup table (sfun) ==
  lookup speed (rad/s) : Inport
  lookup trq (Nm) : Inport  Port=2
  "gear_number  (e.g., 1, 2, 3)" : Inport  Port=3
  Mux : Mux  Inputs=3
  Saturation : Saturate  UpperLimit=max(tx_map_spd)  LowerLimit=min(tx_map_spd)
  Saturation1 : Saturate  UpperLimit=max(tx_map_trq)  LowerLimit=min(tx_map_trq)
  Saturation2 : Saturate  UpperLimit=size(tx_eff_map,3)  LowerLimit=1
  discrete interp2d : S-Function  FunctionName=sfun_discreteLookup3d  Parameters=tx_map_trq, tx_map_spd, tx_eff_map  SFunctionDeploymentMode=off  EnableBusSupport=off
  tx_eff : Outport
  wires:
  discrete interp2d/1 -> tx_eff/1
  Mux/1 -> discrete interp2d/1
  lookup speed (rad/s)/1 -> Saturation/1
  Saturation/1 -> Mux/1
  lookup trq (Nm)/1 -> Saturation1/1
  Saturation1/1 -> Mux/2
  "gear_number  (e.g., 1, 2, 3)"/1 -> Saturation2/1
  Saturation2/1 -> Mux/3

== system BD_PAR_AUTO_base_model/gearbox <gb>/loss (Nm)/Block NOTES ==
  note: 09/20/02:tm modifed lower input to switch after T_loss_at_input to pass the
      | total torque input as the loss when tx_eff=0
      | 5 July 2001:mpo changing loss block to a lookup table methodology
      | 12/20/00:tm revised loss saturation block. lower limit changed
      | from 1 to 0 and upper limit changed from 100 to inf to prevent over or under penalties
  note: Revision Notes:

== system BD_PAR_AUTO_base_model/hydraulic torque converter for  parallel hybrid <htc>/SR/K_adv ==
  "Req'd output trq and spd (Nm), (rad/s)" : Inport
  >0 : Saturate  UpperLimit=inf  LowerLimit=eps
  K_adv=wout/(Tout)^0.5 : Fcn  Expr=u[2]/u[1]^0.5
  Saturation : Saturate  UpperLimit=max(htc_k_adv)  LowerLimit=min(htc_k_adv)
  K_adv : Outport
  wires:
  Saturation/1 -> K_adv/1
  K_adv=wout/(Tout)^0.5/1 -> Saturation/1
  "Req'd output trq and spd (Nm), (rad/s)"/1 -> >0/1
  >0/1 -> K_adv=wout/(Tout)^0.5/1

== system BD_PAR_AUTO_base_model/hydraulic torque converter for  parallel hybrid <htc>/SR/K_adv_coast ==
  "Req'd output trq and spd (Nm), (rad/s)" : Inport
  K_adv=wout/(abs(Tout))^0.5 : Fcn  Expr=u[2]/abs(u[1]+eps)^0.5
  Saturation : Saturate  UpperLimit=max(htc_k_adv_coast)  LowerLimit=0
  K_adv_coast : Outport
  wires:
  "Req'd output trq and spd (Nm), (rad/s)"/1 -> K_adv=wout/(abs(Tout))^0.5/1
  Saturation/1 -> K_adv_coast/1
  K_adv=wout/(abs(Tout))^0.5/1 -> Saturation/1

== system BD_PAR_AUTO_base_model/hydraulic torque converter for  parallel hybrid <htc>/SR/shifting SR ==
  T,w req out : Inport
  w in : Inport  Port=2
  SR : Inport  Port=3
  -3200 rpm/second allowable in engine speed : Gain  Gain=-3200*pi/30  SaturateOnIntegerOverflow=on
  >0 : Saturate  UpperLimit=inf  LowerLimit=eps
  Clock : Clock
  Memory3 : Memory  InitialCondition=eps
  Memory4 : Memory
  MinMax : MinMax  Inputs=2
  SRmax= wout/win,min : Product  Inputs=*/  SaturateOnIntegerOverflow=on
  dt=t-(t-1) : Sum  Inputs=+-  SaturateOnIntegerOverflow=on
  "shifting, then limit  engine speed change" : Switch  Threshold=eps
  win,min= win,prev+rate*dt : Sum  SaturateOnIntegerOverflow=on
  wout,req : Selector  InputPortWidth=2  IndexOptions=Index vector (dialog)  Indices=2  OutputSizes=1
  SR limited : Outport  InitialOutput=0
  wires:
  Memory4/1 -> dt=t-(t-1)/2
  Clock/1 -> Memory4/1, dt=t-(t-1)/1
  dt=t-(t-1)/1 -> -3200 rpm/second allowable in engine speed/1
  Memory3/1 -> win,min= win,prev+rate*dt/1
  win,min= win,prev+rate*dt/1 -> SRmax= wout/win,min/2
  wout,req/1 -> SRmax= wout/win,min/1
  T,w req out/1 -> wout,req/1
  [shifting] -> "shifting, then limit  engine speed change"/2
  SRmax= wout/win,min/1 -> MinMax/1
  SR/1 -> "shifting, then limit  engine speed change"/3, MinMax/2
  "shifting, then limit  engine speed change"/1 -> SR limited/1
  MinMax/1 -> "shifting, then limit  engine speed change"/1
  w in/1 -> >0/1
  >0/1 -> Memory3/1
  -3200 rpm/second allowable in engine speed/1 -> win,min= win,prev+rate*dt/2

== system BD_PAR_AUTO_base_model/hydraulic torque converter for  parallel hybrid <htc>/T, shifting/T_max ==
  w_APU : Inport
  TR : Inport  Port=2
  Block NOTES : Subsystem
      mask Display: disp('Block\nNOTES')
  Constant : Constant
  Gain : Gain  Gain=tc_mc_to_fc_ratio  SaturateOnIntegerOverflow=on
  Gain1 : Gain  Gain=tc_mc_to_fc_ratio  SaturateOnIntegerOverflow=on
  Saturation1 : Saturate  UpperLimit=max(fc_map_spd)*fc_spd_scale  LowerLimit=min(fc_map_spd)*fc_spd_scale
  Sum : Sum  SaturateOnIntegerOverflow=on
  Switch : Switch  Threshold=eps
  Terminator : Terminator
  Tin*TR= Tout : Product  SaturateOnIntegerOverflow=on
  max_torque  mc lookup1 : Lookup  InputValues=mc_map_spd*mc_spd_scale  Table=mc_max_trq*mc_overtrq_factor*mc_trq_scale
  max_torque lookup : Lookup  InputValues=fc_map_spd*fc_spd_scale  Table=fc_max_trq*fc_trq_scale
  T_max max gain from htc : Outport  InitialOutput=0
  wires:
  w_APU/1 -> Saturation1/1
  Tin*TR= Tout/1 -> T_max max gain from htc/1
  TR/1 -> Tin*TR= Tout/2
  max_torque lookup/1 -> Sum/1
  Saturation1/1 -> max_torque lookup/1, Gain/1
  Gain/1 -> max_torque  mc lookup1/1
  max_torque  mc lookup1/1 -> Gain1/1
  Constant/1 -> Switch/2
  Sum/1 -> Switch/1
  Gain1/1 -> Sum/2, Switch/3
  Switch/1 -> Tin*TR= Tout/1
  [engine_on] -> Terminator/1

== system BD_PAR_AUTO_base_model/hydraulic torque converter for  parallel hybrid <htc>/T, shifting/engine speed estimator ==
  htc_spd_in_a : Inport
  Memory2 : Memory
  Out1 : Outport
  wires:
  htc_spd_in_a/1 -> Memory2/1
  Memory2/1 -> Out1/1

== system BD_PAR_AUTO_base_model/mechanical accessory loads <acc>/Mechanical Accessory Loads v2 <acc>/Accessory SDO ==
  data bus : Inport
  Demux : Demux  Outputs=6
      settings: DisplayOption=none
  To Workspace : ToWorkspace  VariableName=acc_mech_trq_r  SampleTime=-1
  To Workspace1 : ToWorkspace  VariableName=acc_mech_pwr_a  SampleTime=-1
  To Workspace2 : ToWorkspace  VariableName=acc_mech_trq_est  SampleTime=-1
  To Workspace3 : ToWorkspace  VariableName=acc_mech_pwr_r  SampleTime=-1
  To Workspace4 : ToWorkspace  VariableName=acc_mech_trq_a  SampleTime=-1
  To Workspace5 : ToWorkspace  VariableName=acc_mech_pwr_est  SampleTime=-1
  mechanical power logging : Subsystem  mask{eff=acc_mech_eff}
      mask prompts: eff "efficiency of accessory systems (decimal)"
  wires:
  Demux/6 -> To Workspace5/1
  Demux/5 -> To Workspace2/1
  Demux/3 -> To Workspace4/1
  Demux/2 -> To Workspace3/1
  Demux/1 -> To Workspace/1
  Demux/4 -> To Workspace1/1, mechanical power logging/1(In1)
  data bus/1 -> Demux/1

== system BD_PAR_AUTO_base_model/mechanical accessory loads <acc>/Mechanical Accessory Loads v2 <acc>/Block NOTES ==
  note: In this model, only one speed is used to predict accessory
      | loading. The forward model is "dummied" out.
  note: A third input is given for accessory load speed. This is done so that
      | the accessory block can use fc_spd_est which is an estimated vehicle speed
      | (equal to fc_spd_out under normal circumstances).
      | Using fc_spd_est provides total compatibility with ADVISOR v3.2
  note: In terms of an interface, the model assumes belt-driven mechanical loads
      | that run off of a prime mover shaft (e.g., engine shaft)
      |
      | This model takes in requested driveline torque and speed requests and
      | augments torque due to belt driven accessories.
      |
      | The torque passed along down to the driveline is only torque to move the
      | vehicle.
  note: This is the mechanical auxiliary loads model.

== system BD_PAR_AUTO_base_model/mechanical accessory loads <acc>/Mechanical Accessory Loads v2 <acc>/backward model ==
  note: Power, W, input to accessory
  note: T, Nm, shaft out
  note: T, Nm, driveline
  note: T, Nm, accessory
  note: w_apu, rad/s
  trq_in : Inport
  spd_in : Inport  Port=2
  acc on/off : Inport  Port=3
  Product : Product  Inputs=**  InputSameDT=on  RndMeth=Zero  SaturateOnIntegerOverflow=on  OutDataTypeStr=Inherit: Same as first input
  Product1 : Product  Inputs=**  InputSameDT=on  RndMeth=Zero  SaturateOnIntegerOverflow=on  OutDataTypeStr=Inherit: Same as first input
  Sum : Sum  Inputs=|++  InputSameDT=on  SaturateOnIntegerOverflow=on  OutDataTypeStr=Inherit: Same as first input
  acc_mech_var_loads : ToWorkspace  VariableName=acc_mech_var_load  SaveFormat=Structure  SampleTime=-1
  mechanical accessories (Nm) : Subsystem  BlockChoice=Mechanical Accessories: Const Mech Var Elect
      settings: AttributesFormatString=%<BlockChoice>  TemplateBlock=lib_accessory/mechanical accessories (Nm)  MemberBlocks=Mechanical Accessories: Const Mech Var Elect,Mechanical Accessories: Constant Mechanical & Electrical,Mechanical Accessories: Speed Dependant and Variable Electrical,Saber Dual Voltage Cosim,Saber Single Voltage Cosim,SindaTransAC
      mask Display: image(imread('bdi_acc_pic_cs.bmp'))
  trq_out : Outport
  acc_mech_trq_r : Outport  Port=2
  acc_mech_pwr_r : Outport  Port=3
  wires:
  mechanical accessories (Nm)/3(probes) -> acc_mech_var_loads/1
  [acc_on] -> Product1/2
  [acc_on] -> Product/1
  acc on/off/1 -> [acc_on]
  mechanical accessories (Nm)/2(P_mech_acc) -> Product1/1
  Product1/1 -> acc_mech_pwr_r/1
  mechanical accessories (Nm)/1(T_acc) -> Product/2
  Product/1 -> Sum/2, acc_mech_trq_r/1
  Sum/1 -> trq_out/1
  trq_in/1 -> Sum/1
  spd_in/1 -> mechanical accessories (Nm)/1(w_APU)

== system BD_PAR_AUTO_base_model/mechanical accessory loads <acc>/Mechanical Accessory Loads v2 <acc>/forward model ==
  note: acc torque, Nm
  note: NOTES
  note: This simplistic model may not correctly account for accessory torque and/or power
      | when the upstream torque provider is torque or speed limited
  note: Power, W, input to accessory
  note: T, Nm, shaft out
  note: driveline and
      | acc torque, Nm
  note: T, Nm, accessory
  note: acc speed, rad/s
  trq_in : Inport
  spd_in : Inport  Port=2
  acc_trq_req : Inport  Port=3
  Product1 : Product  Inputs=**  InputSameDT=on  RndMeth=Zero  SaturateOnIntegerOverflow=on  OutDataTypeStr=Inherit: Same as first input
  Sum : Sum  Inputs=|+-  InputSameDT=on  SaturateOnIntegerOverflow=on  OutDataTypeStr=Inherit: Same as first input
  trq_out : Outport
  acc_mech_trq_a : Outport  Port=2
  acc_mech_pwr_a : Outport  Port=3
  wires:
  [pm_trq_a] -> Sum/1
  acc_trq_req/1 -> [acc_trq_r]
  trq_in/1 -> [pm_trq_a]
  [acc_spd] -> Product1/2
  [acc_trq_r] -> Product1/1, Sum/2, acc_mech_trq_a/1
  Product1/1 -> acc_mech_pwr_a/1
  Sum/1 -> trq_out/1
  spd_in/1 -> [acc_spd]
